simulink model "stateflow6"  (R2015a)
settings: Solver=ode3  StartTime=0.0  StopTime=inf  RelTol=1e-3
values from neighbouring files (symbols this model uses):
  ObjCarGapMax = 20    [initial.m]
  ObjCarGapMin = 4    [initial.m]
  ObjLengthMax = 35    [initial.m]
  ObjLengthMin = 25    [initial.m]
  ObjUltrSnsrOffset = 2    [initial.m]
  ParkCarDepthMax = 40    [initial.m]
  ParkCarDepthMin = 24    [initial.m]
  ParkLengthMax = 46    [initial.m]
  ParkLengthMin = 35    [initial.m]
  ParkUltrSnsrOffset = 5    [initial.m]
undefined symbols (not defined in the file or in its folder): sigbuilder_block
libraries: legoev3lib x6
settings Model: SimulationMode=external  ExtModeTrigDuration=2  Creator=Keshav  LastModifiedBy=Keshav
settings OptimizationCC: OptimizeModelRefInitCode=on  LifeSpan=1
settings DebuggingCC: UnderspecifiedInitializationDetection=Classic  MergeDetectMultiDrivingBlocksExec=none
settings HardwareCC: ProdLargestAtomicInteger=Long  ProdLargestAtomicFloat=Float  ProdEndianess=LittleEndian  ProdHWDeviceType=ARM Compatible->ARM 9
settings RTWCC: SystemTargetFile=realtime.tlc  GenerateMakefile=off  TemplateMakefile=realtime.tmf  Description=Run on Target Hardware  RTWVerbose=off
settings ERTTargetCC: CombineOutputUpdateFcns=off  ERTSrcFileBannerTemplate=realtime_code_template.cgt  ERTHdrFileBannerTemplate=realtime_code_template.cgt  ERTDataSrcFileTemplate=realtime_code_template.cgt  ERTDataHdrFileTemplate=realtime_code_template.cgt  ERTCustomFileTemplate=realtime_file_process.tlc

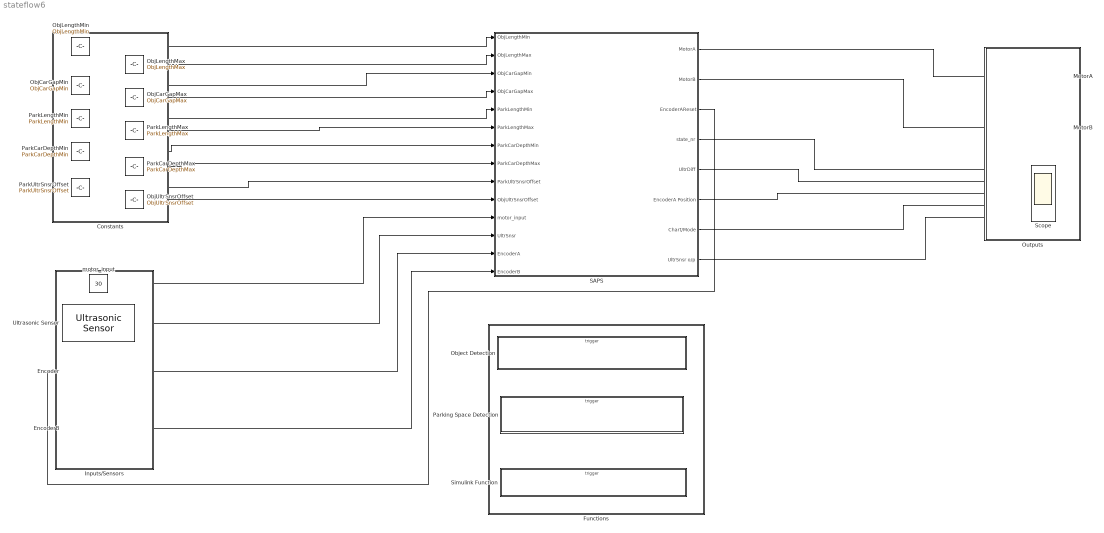
== system stateflow6 ==
  Constants : Subsystem
  Encoder : legoev3lib/Encoder  portNumber=A  opMode=Reset by external signal  sampleTime=0.01
  EncoderB : legoev3lib/Encoder  portNumber=B  opMode=No reset  sampleTime=0.01
  Functions : Subsystem
  Inputs/Sensors : Subsystem
  MotorA : legoev3lib/Motor  sportNumber=A  sstopAction=Brake
  MotorB : legoev3lib/Motor  sportNumber=B  sstopAction=Brake
  ObjCarGapMax : Constant  Value=ObjCarGapMax
  ObjCarGapMin : Constant  Value=ObjCarGapMin
  ObjLengthMax : Constant  Value=ObjLengthMax
  ObjLengthMin : Constant  Value=ObjLengthMin
  ObjUltrSnsrOffset : Constant  Value=ObjUltrSnsrOffset
  Object Detection : Subsystem  TreatAsAtomicUnit=on
  Outputs : Subsystem
  ParkCarDepthMax : Constant  Value=ParkCarDepthMax
  ParkCarDepthMin : Constant  Value=ParkCarDepthMin
  ParkLengthMax : Constant  Value=ParkLengthMax
  ParkLengthMin : Constant  Value=ParkLengthMin
  ParkUltrSnsrOffset : Constant  Value=ParkUltrSnsrOffset
  Parking Space Detection : Subsystem  TreatAsAtomicUnit=on
  SAPS : Subsystem
  Scope : Scope  NumInputPorts=5
      settings: TimeRange=9.76  YMin=1~-20~0~1~0  YMax=2~20~60~2~40  SaveName=ScopeData4
  Simulink Function : Subsystem  TreatAsAtomicUnit=on
  Ultrasonic Sensor : legoev3lib/Ultrasonic Sensor  PortNumber=1  sampleTime=0.01
  motor_input : Constant  Value=30
  wires:
  ObjLengthMin/1 -> SAPS/1(ObjLengthMin)
  ObjLengthMax/1 -> SAPS/2(ObjLengthMax)
  ObjCarGapMin/1 -> SAPS/3(ObjCarGapMin)
  ObjCarGapMax/1 -> SAPS/4(ObjCarGapMax)
  ParkLengthMin/1 -> SAPS/5(ParkLengthMin)
  ParkLengthMax/1 -> SAPS/6(ParkLengthMax)
  ParkCarDepthMin/1 -> SAPS/7(ParkCarDepthMin)
  ParkCarDepthMax/1 -> SAPS/8(ParkCarDepthMax)
  ParkUltrSnsrOffset/1 -> SAPS/9(ParkUltrSnsrOffset)
  ObjUltrSnsrOffset/1 -> SAPS/10(ObjUltrSnsrOffset)
  motor_input/1 -> SAPS/11(motor_input)
  Ultrasonic Sensor/1 -> SAPS/12(UltrSnsr)
  Encoder/1 -> SAPS/13(EncoderA)
  SAPS/1(MotorA) -> MotorA/1
  SAPS/3(EncoderAReset) -> Encoder/1
  SAPS/4(state_nr) -> Scope/1
  SAPS/5(UltrDiff) -> Scope/2
  SAPS/6(EncoderA Position) -> Scope/3
  SAPS/7(Chart/Mode) -> Scope/4
  SAPS/8(UltrSnsr o/p) -> Scope/5
  SAPS/2(MotorB) -> MotorB/1
  EncoderB/1 -> SAPS/14(EncoderB)

== system stateflow6/Constants ==

== system stateflow6/Functions ==

== system stateflow6/Inputs//Sensors ==

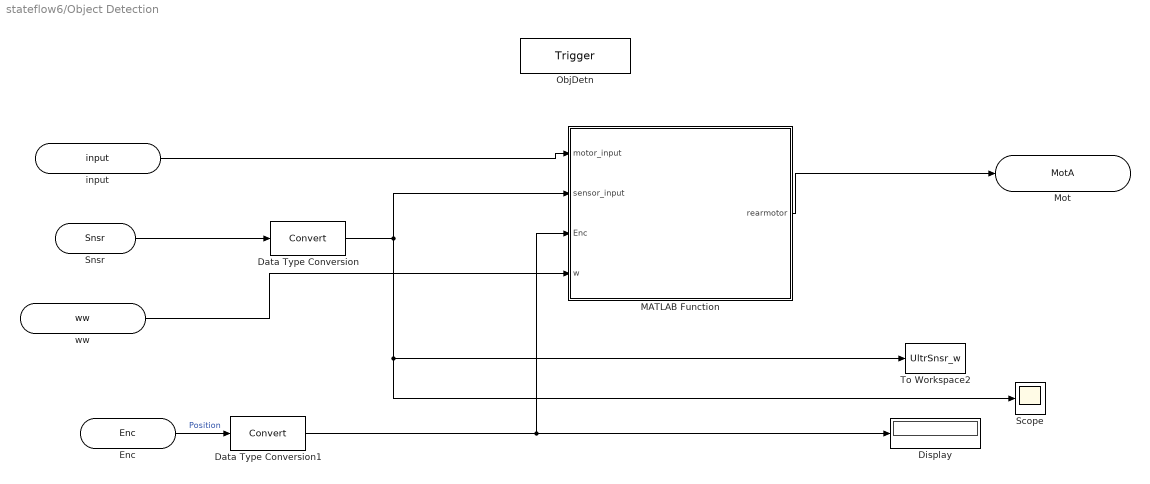
== system stateflow6/Object Detection ==
  ObjDetn : TriggerPort  TriggerType=function-call  IsSimulinkFunction=on  FunctionName=ObjDetn
  Data Type Conversion : DataTypeConversion
  Data Type Conversion1 : DataTypeConversion
  Display : Display
  MATLAB Function : MATLAB Function  TreatAsAtomicUnit=on
  Scope : Scope
      settings: YMin=2.85  YMax=3.15
  To Workspace2 : ToWorkspace  VariableName=UltrSnsr_w  SampleTime=-1
  input : ArgIn  DisableCoverage=on  ArgumentName=input
  Snsr : ArgIn  DisableCoverage=on  Port=2  ArgumentName=Snsr
  Enc : ArgIn  DisableCoverage=on  Port=3  ArgumentName=Enc
  ww : ArgIn  DisableCoverage=on  Port=4  ArgumentName=ww
  Mot : ArgOut  DisableCoverage=on  ArgumentName=MotA
  wires:
  Data Type Conversion/1 -> To Workspace2/1, Scope/1, MATLAB Function/2(sensor_input)
  MATLAB Function/1(rearmotor) -> Mot/1
  Enc/1 -> Data Type Conversion1/1  "Position"
  Snsr/1 -> Data Type Conversion/1
  input/1 -> MATLAB Function/1(motor_input)
  Data Type Conversion1/1 -> Display/1, MATLAB Function/3(Enc)
  ww/1 -> MATLAB Function/4(w)

== system stateflow6/Outputs ==

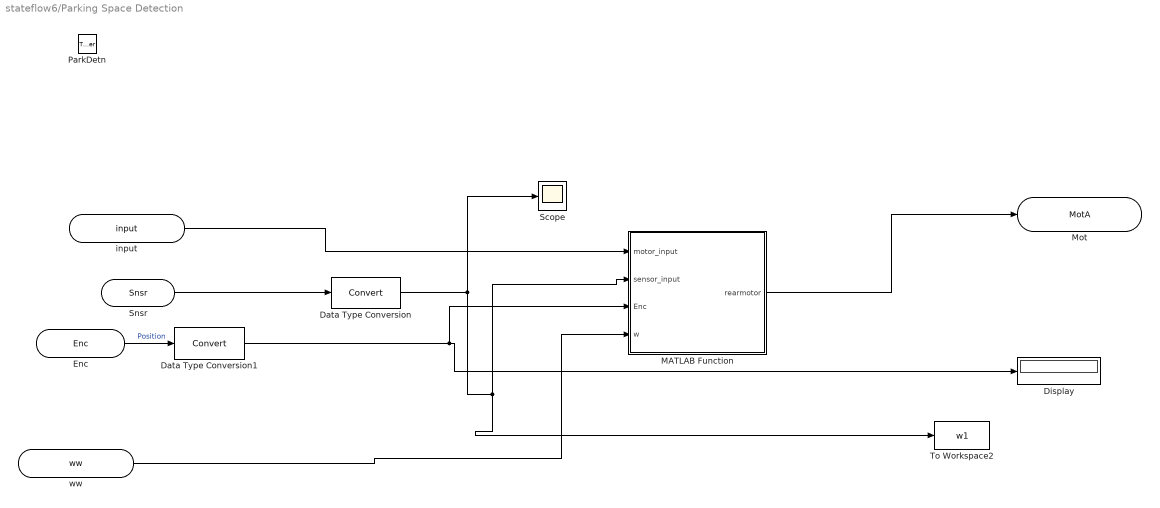
== system stateflow6/Parking Space Detection ==
  ParkDetn : TriggerPort  TriggerType=function-call  IsSimulinkFunction=on  FunctionName=ParkDetn
  Data Type Conversion : DataTypeConversion
  Data Type Conversion1 : DataTypeConversion
  Display : Display
  MATLAB Function : MATLAB Function  TreatAsAtomicUnit=on
  Scope : Scope
      settings: YMin=3  YMax=3
  To Workspace2 : ToWorkspace  VariableName=w1  SampleTime=-1
  input : ArgIn  DisableCoverage=on  ArgumentName=input
  Snsr : ArgIn  DisableCoverage=on  Port=2  ArgumentName=Snsr
  Enc : ArgIn  DisableCoverage=on  Port=3  ArgumentName=Enc
  ww : ArgIn  DisableCoverage=on  Port=4  ArgumentName=ww
  Mot : ArgOut  DisableCoverage=on  ArgumentName=MotA
  wires:
  Data Type Conversion/1 -> To Workspace2/1, MATLAB Function/2(sensor_input), Scope/1
  MATLAB Function/1(rearmotor) -> Mot/1
  Enc/1 -> Data Type Conversion1/1  "Position"
  Snsr/1 -> Data Type Conversion/1
  input/1 -> MATLAB Function/1(motor_input)
  Data Type Conversion1/1 -> MATLAB Function/3(Enc), Display/1
  ww/1 -> MATLAB Function/4(w)

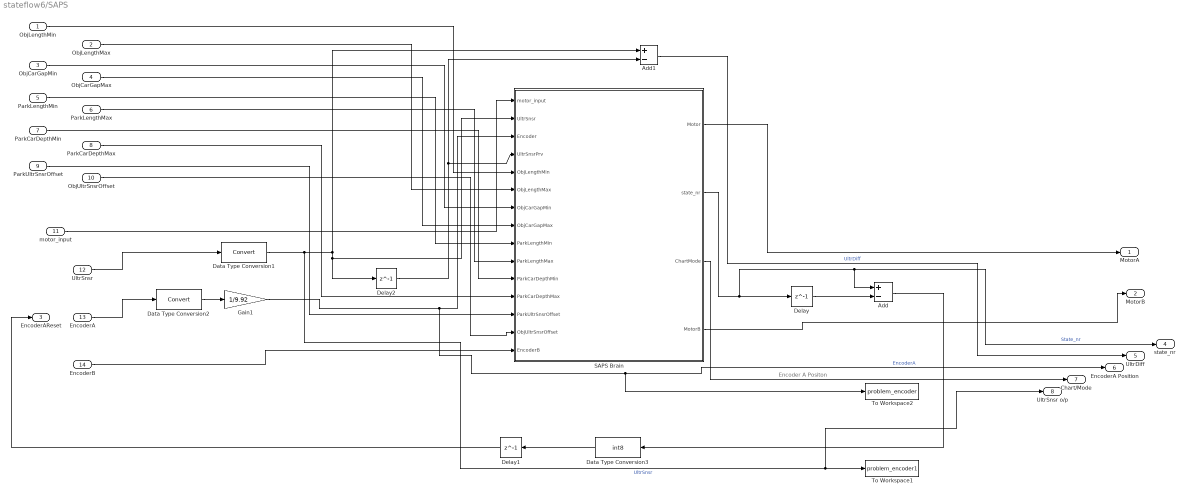
== system stateflow6/SAPS ==
  note: Encoder A Positon
  ObjLengthMin : Inport
  ObjLengthMax : Inport  Port=2
  ObjCarGapMin : Inport  Port=3
  ObjCarGapMax : Inport  Port=4
  ParkLengthMin : Inport  Port=5
  ParkLengthMax : Inport  Port=6
  ParkCarDepthMin : Inport  Port=7
  ParkCarDepthMax : Inport  Port=8
  ParkUltrSnsrOffset : Inport  Port=9
  ObjUltrSnsrOffset : Inport  Port=10
  motor_input : Inport  Port=11
  UltrSnsr : Inport  Port=12
  EncoderA : Inport  Port=13
  EncoderB : Inport  Port=14
  Add : Sum  Inputs=+-
  Add1 : Sum  Inputs=+-
  Data Type Conversion1 : DataTypeConversion
  Data Type Conversion2 : DataTypeConversion
  Data Type Conversion3 : DataTypeConversion  OutDataTypeStr=int8
  Delay : Delay  DelayLength=1  InitialCondition=0
  Delay1 : Delay  DelayLength=1  InitialCondition=0
  Delay2 : Delay  DelayLength=1  InitialCondition=0
  Gain1 : Gain  Gain=1/9.92
  SAPS Brain : Stateflow chart  TreatAsAtomicUnit=on
  To Workspace1 : ToWorkspace  VariableName=problem_encoder1  SampleTime=-1
  To Workspace2 : ToWorkspace  VariableName=problem_encoder  SampleTime=-1
  MotorA : Outport
  MotorB : Outport  Port=2
  EncoderAReset : Outport  Port=3
  state_nr : Outport  Port=4
  UltrDiff : Outport  Port=5
  EncoderA Position : Outport  Port=6
  Chart/Mode : Outport  Port=7
  UltrSnsr o/p : Outport  Port=8
  wires:
  Data Type Conversion1/1 -> SAPS Brain/2(UltrSnsr), Delay2/1, Add1/1, UltrSnsr o/p/1, To Workspace1/1  "UltrSnsr"
  Data Type Conversion2/1 -> Gain1/1
  UltrSnsr/1 -> Data Type Conversion1/1
  motor_input/1 -> SAPS Brain/1(motor_input)
  SAPS Brain/1(Motor) -> MotorA/1
  EncoderA/1 -> Data Type Conversion2/1
  Add/1 -> Data Type Conversion3/1
  Gain1/1 -> SAPS Brain/3(Encoder), EncoderA Position/1, To Workspace2/1  "EncoderA"
  SAPS Brain/2(state_nr) -> state_nr/1, Add/1, Delay/1  "State_nr"
  Delay/1 -> Add/2
  Data Type Conversion3/1 -> Delay1/1
  ObjCarGapMin/1 -> SAPS Brain/7(ObjCarGapMin)
  SAPS Brain/3(ChartMode) -> Chart/Mode/1
  Delay2/1 -> Add1/2, SAPS Brain/4(UltrSnsrPrv)
  Add1/1 -> UltrDiff/1  "UltrDiff"
  Delay1/1 -> EncoderAReset/1
  ObjLengthMin/1 -> SAPS Brain/5(ObjLengthMin)
  ObjLengthMax/1 -> SAPS Brain/6(ObjLengthMax)
  ObjCarGapMax/1 -> SAPS Brain/8(ObjCarGapMax)
  ParkLengthMin/1 -> SAPS Brain/9(ParkLengthMin)
  ParkLengthMax/1 -> SAPS Brain/10(ParkLengthMax)
  ParkCarDepthMin/1 -> SAPS Brain/11(ParkCarDepthMin)
  ParkCarDepthMax/1 -> SAPS Brain/12(ParkCarDepthMax)
  ParkUltrSnsrOffset/1 -> SAPS Brain/13(ParkUltrSnsrOffset)
  ObjUltrSnsrOffset/1 -> SAPS Brain/14(ObjUltrSnsrOffset)
  SAPS Brain/4(MotorB) -> MotorB/1
  EncoderB/1 -> SAPS Brain/15(EncoderB)

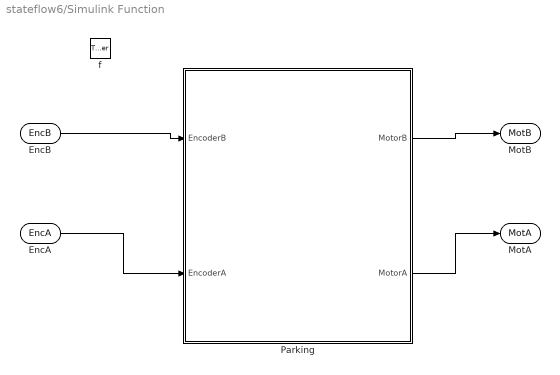
== system stateflow6/Simulink Function ==
  f : TriggerPort  TriggerType=function-call  IsSimulinkFunction=on  FunctionName=f
  Parking : Subsystem
  EncB : ArgIn  DisableCoverage=on  ArgumentName=EncB
  EncA : ArgIn  DisableCoverage=on  Port=2  ArgumentName=EncA
  MotB : ArgOut  DisableCoverage=on  ArgumentName=MotB
  MotA : ArgOut  DisableCoverage=on  Port=2  ArgumentName=MotA
  wires:
  EncB/1 -> Parking/1(EncoderB)
  Parking/1(MotorB) -> MotB/1
  Parking/2(MotorA) -> MotA/1
  EncA/1 -> Parking/2(EncoderA)

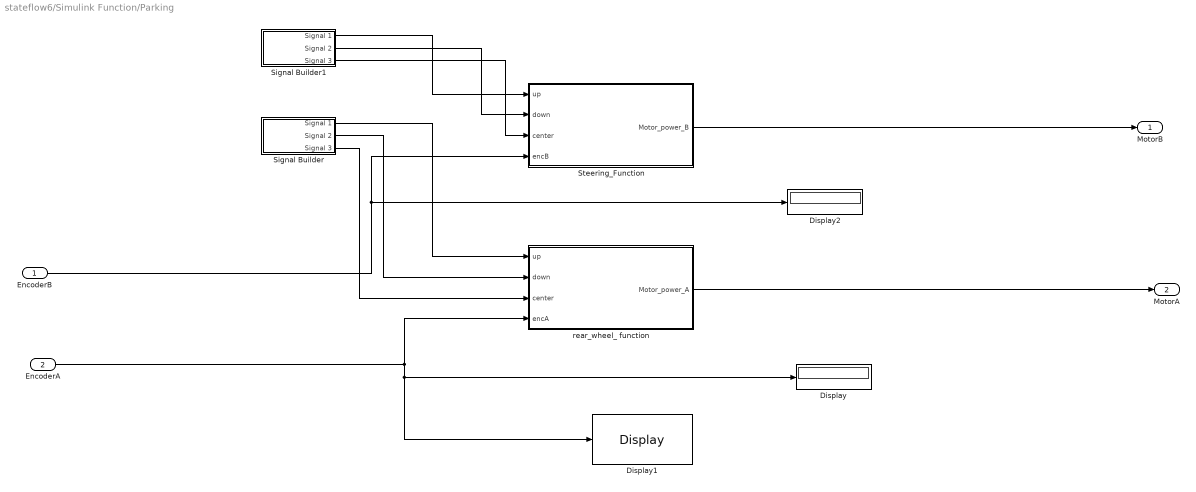
== system stateflow6/Simulink Function/Parking ==
  EncoderB : Inport
  EncoderA : Inport  Port=2
  " Steering_Function" : MATLAB Function  TreatAsAtomicUnit=on
  Display : Display
      settings: Format=decimal (Stored Integer)
  Display1 : legoev3lib/Display  slcdStr=enc A  slcdLine=1  slcdFormat=Decimal
  Display2 : Display
      settings: Format=decimal (Stored Integer)
  Signal Builder : Subsystem  Tag=STV Subsys  LoadFcn=sigbuilder_block('load');  StartFcn=sigbuilder_block('start');  StopFcn=sigbuilder_block('stop');  ClipboardFcn=sigbuilder_block('clipboard');  mask(Sigbuilder block){}
      mask help: Simulink:masks:SigbuilderBlock_MD
      mask init:
      | if ~strcmp(get_param(bdroot(gcbh),'SimulationStatus'),'stopped') tuvar = sigbuilder_block('maskInit'); end
      settings: CopyFcn=sigbuilder_block('copy');  DeleteFcn=sigbuilder_block('delete');  ModelCloseFcn=sigbuilder_block('modelClose');  PreSaveFcn=sigbuilder_block('preSave');  PauseFcn=sigbuilder_block('pause');  ContinueFcn=sigbuilder_block('continue');  NameChangeFcn=sigbuilder_block('namechange');  OpenFcn=sigbuilder_block('open',[438 199 636 400 ]);  CloseFcn=sigbuilder_block('close');
      mask Display: plot(0, 0, 100, 100,[2, 2, 32, 32, 2], [68, 8, 8, 68, 68],[32, 2], [38, 38], [32, 19, 2],[53, 60, 44], [32, 17, 17, 2],[16, 16, 31, 31]);txt = getActiveGroup(gcbh);text(2, 100, txt,'verticalAlignment', 'top');
  Signal Builder1 : Subsystem  Tag=STV Subsys  LoadFcn=sigbuilder_block('load');  StartFcn=sigbuilder_block('start');  StopFcn=sigbuilder_block('stop');  ClipboardFcn=sigbuilder_block('clipboard');  mask(Sigbuilder block){}
      mask help: Simulink:masks:SigbuilderBlock_MD
      mask init:
      | if ~strcmp(get_param(bdroot(gcbh),'SimulationStatus'),'stopped') tuvar = sigbuilder_block('maskInit'); end
      settings: CopyFcn=sigbuilder_block('copy');  DeleteFcn=sigbuilder_block('delete');  ModelCloseFcn=sigbuilder_block('modelClose');  PreSaveFcn=sigbuilder_block('preSave');  PauseFcn=sigbuilder_block('pause');  ContinueFcn=sigbuilder_block('continue');  NameChangeFcn=sigbuilder_block('namechange');  OpenFcn=sigbuilder_block('open',[438 199 636 400 ]);  CloseFcn=sigbuilder_block('close');
      mask Display: plot(0, 0, 100, 100,[2, 2, 32, 32, 2], [68, 8, 8, 68, 68],[32, 2], [38, 38], [32, 19, 2],[53, 60, 44], [32, 17, 17, 2],[16, 16, 31, 31]);txt = getActiveGroup(gcbh);text(2, 100, txt,'verticalAlignment', 'top');
  rear_wheel_ function : MATLAB Function  TreatAsAtomicUnit=on
  MotorB : Outport
  MotorA : Outport  Port=2
  wires:
  " Steering_Function"/1(Motor_power_B) -> MotorB/1
  Signal Builder1/3(Signal 3) -> " Steering_Function"/3(center)
  rear_wheel_ function/1(Motor_power_A) -> MotorA/1
  Signal Builder/3(Signal 3) -> rear_wheel_ function/3(center)
  Signal Builder1/1(Signal 1) -> " Steering_Function"/1(up)
  Signal Builder/2(Signal 2) -> rear_wheel_ function/2(down)
  EncoderA/1 -> Display1/1, Display/1, rear_wheel_ function/4(encA)
  Signal Builder1/2(Signal 2) -> " Steering_Function"/2(down)
  Signal Builder/1(Signal 1) -> rear_wheel_ function/1(up)
  EncoderB/1 -> " Steering_Function"/4(encB), Display2/1

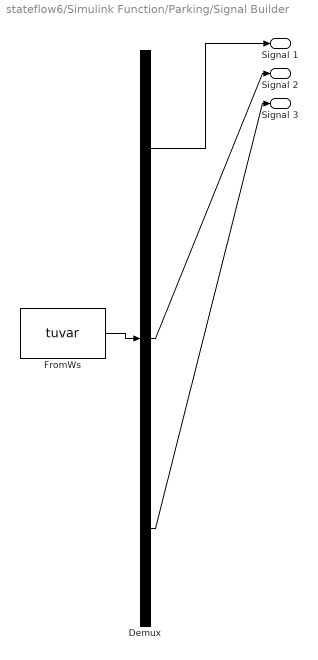
== system stateflow6/Simulink Function/Parking/Signal Builder ==
  Demux : Demux  Tag=STV Demux  Outputs=3
  FromWs : FromWorkspace  Tag=STV FromWs  VariableName=tuvar  SampleTime=0
      SigBuilderData=|
      | common.afterFinalStr = 'Extrapolate'
      | common.sampleTime = 0
      | dataSet.timeRange = [0 20]
      | dataSet.name = 'Move'
      | sbobj.Groups.Name = 'Move'
      | sbobj.Groups.Signals(1).Name = 'Signal 1'
      | sbobj.Groups.Signals(1).XData = [0 2 2 5 5 20]
      | sbobj.Groups.Signals(1).YData = [0 0 1 1 0 0]
      | sbobj.Groups.Signals(2).Name = 'Signal 2'
      | sbobj.Groups.Signals(2).XData = [0 7.1 7.1 10 10 20]
      | sbobj.Groups.Signals(2).YData = [0 0 1 1 0 0]
      | sbobj.Groups.Signals(3).Name = 'Signal 3'
      | sbobj.Groups.Signals(3).XData = [0 12.75 12.75 15.95 15.95 20]
      | sbobj.Groups.Signals(3).YData = [0 0 1 1 0 0]
      | sbobj.Groups.TimeRange = [0 20]
  Signal 1 : Outport  Tag=STV Outport
  Signal 2 : Outport  Tag=STV Outport  Port=2
  Signal 3 : Outport  Tag=STV Outport  Port=3
  wires:
  Demux/1 -> Signal 1/1
  FromWs/1 -> Demux/1
  Demux/2 -> Signal 2/1
  Demux/3 -> Signal 3/1

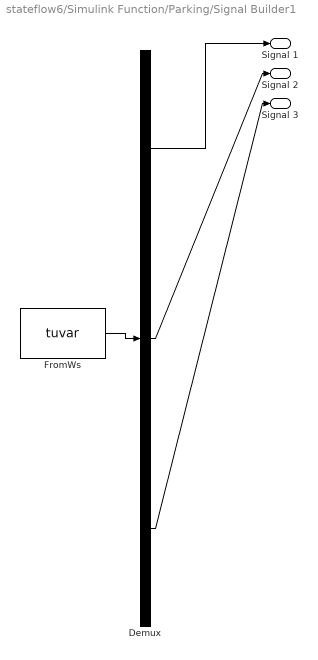
== system stateflow6/Simulink Function/Parking/Signal Builder1 ==
  Demux : Demux  Tag=STV Demux  Outputs=3
  FromWs : FromWorkspace  Tag=STV FromWs  VariableName=tuvar  SampleTime=0
      SigBuilderData=|
      | common.afterFinalStr = 'Extrapolate'
      | common.sampleTime = 0
      | dataSet.timeRange = [0 20]
      | dataSet.name = 'Steering'
      | sbobj.Groups.Name = 'Steering'
      | sbobj.Groups.Signals(1).Name = 'Signal 1'
      | sbobj.Groups.Signals(1).XData = [0 0.12 0.12 2.02 2.02 20]
      | sbobj.Groups.Signals(1).YData = [0 0 1 1 0 0]
      | sbobj.Groups.Signals(2).Name = 'Signal 2'
      | sbobj.Groups.Signals(2).XData = [0 5 5 7 7 20]
      | sbobj.Groups.Signals(2).YData = [0 0 1 1 0 0]
      | sbobj.Groups.Signals(3).Name = 'Signal 3'
      | sbobj.Groups.Signals(3).XData = [0 10 10 12 12 20]
      | sbobj.Groups.Signals(3).YData = [0 0 1 1 0 0]
      | sbobj.Groups.TimeRange = [0 20]
  Signal 1 : Outport  Tag=STV Outport
  Signal 2 : Outport  Tag=STV Outport  Port=2
  Signal 3 : Outport  Tag=STV Outport  Port=3
  wires:
  Demux/2 -> Signal 2/1
  FromWs/1 -> Demux/1
  Demux/1 -> Signal 1/1
  Demux/3 -> Signal 3/1

== matlab function stateflow6/Parking Space Detection/MATLAB Function ==
  data: motor_input input; sensor_input input; Enc input; rearmotor output; w input
function rearmotor = fcn(motor_input,sensor_input,Enc,w)
%#codegen
%d = z
%u = 0; %Encoder reset
% x = w;
% length2=0;
%reset11=0;
%state3=0;
if(sensor_input>ParkCarDepthMin)&&(sensor_input<=ParkCarDepthMax)
    rearmotor=motor_input-10;
%     if((sensor_input-w)>2)||((sensor_input-w)<-2)
%         rearmotor = motor_input - 15;
%     elseif(sensor_input>4)&&(sensor_input<=20)
%         rearmotor = motor_input-15;
%      end

  %  if (Enc>=73)&&(Enc<=74)
   %     length2=Enc;
 %       rearmotor=0;
%        reset11=1;
    %    state3=1;        
    %end
    %elseif(sensor_input>20)&&(sensor_input<=35)
 %   rearmotor=motor_input;
%else(sensor_input>24)&&(sensor_input<=61)
 %   x = u;
  %  rearmotor=motor_input-10;
   % u=1;    
    %if(sensor_input<=20)
    %    rearmotor=0;   
%else((sensor_input-z)>2)||((sensor_input-z)<-2)
   % rearmotor=0;
else
    rearmotor = motor_input - 10;

%state3=0;
end



end

== matlab function stateflow6/Object Detection/MATLAB Function ==
  data: motor_input input; sensor_input input; rearmotor output; Enc input; w input
function rearmotor = fcn(motor_input,sensor_input,Enc,w)
%#codegen
%d = z
%u = 0; %Encoder reset
%x = w;
%lenght=0;
%reset1=0;
%state2=0;
if(sensor_input>ObjCarGapMin)&&(sensor_input<=ObjCarGapMax)
    rearmotor=motor_input;
%     if((sensor_input-w)>2)|| ((sensor_input-w)<-2)
%         rearmotor = motor_input - 15;
%     elseif(sensor_input>4)&&(sensor_input<=20)
%         rearmotor = motor_input-5;
%     end
%    if (Enc>=30)&&(Enc<=32)
 %       length1=30;
%        rearmotor=0;
%        reset1=1;
     %   state2=1;        
  %  end
    %elseif(sensor_input>20)&&(sensor_input<=35)
 %   rearmotor=motor_input;
%else(sensor_input>24)&&(sensor_input<=61)
 %   x = u;
  %  rearmotor=motor_input-10;
   % u=1;    
    %if(sensor_input<=20)
    %    rearmotor=0;   
%else((sensor_input-z)>2)||((sensor_input-z)<-2)
   % rearmotor=0;
else
    rearmotor = motor_input - 10;
    %state2=0;
end



end

== stateflow chart stateflow6/SAPS/SAPS Brain ==
  state First_Object
    en:
    state_nr=1;
    du:
    Motor = ObjDetn(motor_input,UltrSnsr,Encoder,w);
  note: 
  note: 
  state Parking
    en:
    state_nr=4;
    du:
    [Motor,MotorB] = f(EncB,Encoder);
  state Park_Space
    en:
    state_nr=2;
    du:
    Motor = ParkDetn(motor_input,UltrSnsr,Encoder,w);
    note: 
    note: 
  state Second_Object
    en:
    state_nr=3;
    du:
    Motor = ObjDetn(motor_input,UltrSnsr,Encoder,w);
    ex:
    Motor=0;
  (default) -> First_Object
  (junction 160) -> First_Object
  First_Object -> (junction 160) [order 1] : after(100, msec)
      | [(UltrSnsr-UltrSnsrPrv)>ObjUltrSnsrOffset || (UltrSnsr-UltrSnsrPrv)<-ObjUltrSnsrOffset && Encoder<ObjLengthMin]
  Second_Object -> (junction 160) [order 2] : after(100, msec)
      | [(UltrSnsr-UltrSnsrPrv)>ObjUltrSnsrOffset || (UltrSnsr-UltrSnsrPrv)<-ObjUltrSnsrOffset && Encoder<ObjLengthMin]
  Park_Space -> (junction 160) [order 1] : after(100, msec)
      | [(UltrSnsr-UltrSnsrPrv)>ParkUltrSnsrOffset || (UltrSnsr-UltrSnsrPrv)<-ParkUltrSnsrOffset && Encoder<ParkLengthMin]
  First_Object -> Park_Space [order 2] : [UltrSnsr>=ParkCarDepthMin && UltrSnsr<=ParkCarDepthMax && Encoder>=ObjLengthMin && Encoder<=ObjLengthMax]
  Second_Object -> Parking [order 1] : [UltrSnsr>=ObjCarGapMin && UltrSnsr<=ObjCarGapMax && Encoder>=ObjLengthMin && Encoder<=ObjLengthMax]
  Park_Space -> Second_Object [order 2] : [UltrSnsr>ObjCarGapMin && UltrSnsr<=ObjCarGapMax && Encoder>=ParkLengthMin && Encoder<=ParkLengthMax]
  data: motor_input input; Motor output; UltrSnsr input; Encoder input; state_nr output; UltrSnsrPrv input; ChartMode output Enum: ChartModeType; ObjLengthMin input; ObjLengthMax input; ObjCarGapMin input; ObjCarGapMax input; ParkLengthMin input; ParkLengthMax input; ParkCarDepthMin input; ParkCarDepthMax input; ParkUltrSnsrOffset input; ObjUltrSnsrOffset input; MotorB output; EncoderB input

== matlab function stateflow6/Simulink Function/Parking/ Steering_Function ==
  data: up input; down input; center input; Motor_power_B output; encB input
function Motor_power_B=fcn(up,down,center,encB)
%#codegen
if(up==1)&&(encB>=-400)
   Motor_power_B=-70;
elseif(down==1)&&(encB<=400)
   Motor_power_B=70;
elseif (center==1)&&(encB>=5)
 %%  while(encB~=0)
   Motor_power_B=-70;
else
   Motor_power_B=0;
end
end

== matlab function stateflow6/Simulink Function/Parking/rear_wheel_ function ==
  data: Motor_power_A output; up input; down input; center input; encA input
function Motor_power_A=fcn(up, down,center,encA)
%#codegen
if (up==1)&&(encA>=-240)
  Motor_power_A = -30;
elseif (down==1)&&(encA>=-500)
     Motor_power_A = -30;
elseif (center==1)&&(encA<=-445)
    Motor_power_A=30;
else
    Motor_power_A=0; 
end
end
